simulink model "visodo10"  (Simulink 7.5)
settings: Solver=FixedStepDiscrete  StartTime=0.0  StopTime=220  FixedStep=1  RelTol=1e-3
undefined symbols (not defined in the file): gray, strel
libraries: vipsnks x2, viptextngfix x1, vipmorphops x1
(part 1 of 2)
settings Model: Creator=jfabia02  LastModifiedBy=jfabia02  SimulationMode=external  ExtModeEnableFloating=off  ExtModeArchiveFileName=model_output  ExtModeArchiveDirName=C:\RTtools\VU-RLNX\RLNX\RLNX\Simulink Models
settings RTWCC: SystemTargetFile=rlnx.tlc  GenCodeOnly=on  TemplateMakefile=rlnx_ubuntu.tmf  Description=Linux Real-Time Target  ProcessScript=rlnx_make_rtw_hook
settings CodeAppCC: GenerateComments=off  SimulinkBlockComments=off
settings STFCustomTargetCC: TargetFunctionLibrary=GNU99 (GNU)  ModelReferenceCompliant=off  GeneratePreprocessorConditionals=Disable all  MatFileLogging=on  SystemTargetFile=rlnx.tlc
settings GRTTargetCC: TargetFunctionLibrary=GNU99 (GNU)  ModelReferenceCompliant=off  ParMdlRefBuildCompliant=off  CompOptLevelCompliant=off  ExtMode=on  ExtModeMexArgs='10.0.0.1'
settings CustomProperty: DataType=string  Value=-lm -ldl /matlab_includes/libfreenect/build/lib/libfreenect.so.0.0.1
settings EnumStrPairs: String=PC

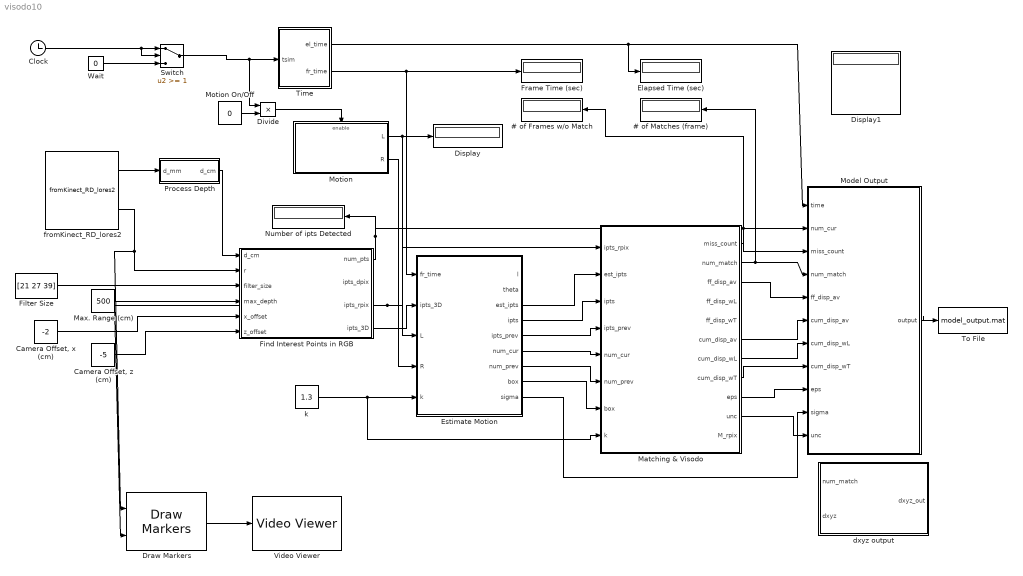
== system visodo10 ==
  # of Frames w/o Match : Display
  # of Matches (frame) : Display
  "Camera Offset, x (cm)" : Constant  Value=-2  OutDataTypeMode=double  OutDataType=fixdt(1, 16)  OutScaling=2^0  OutDataTypeStr=double
  "Camera Offset, z (cm)" : Constant  Value=-5  OutDataTypeMode=double  OutDataType=fixdt(1, 16)  OutScaling=2^0  OutDataTypeStr=double
  Clock : Clock
      settings: Decimation=10
  Display : Display
  Display1 : Display
  Divide : Product  Inputs=**  OutDataType=fixdt(1, 16)  OutScaling=2^-10
  Draw Markers : viptextngfix/Draw Markers  DialogController=vipDDGCreate  DialogControllerArgs=DataTag0  shape=Circle  size=3  fill=off  fillClrSource=Specify via dialog  display=Black  intensity=200  color=[200 255 100]  opacity=0.6  viewport=Entire image  antialiasing=off  inType=Obsolete  imagePorts=One multidimensional signal  prodOutputMode=Binary point scaling  prodOutputWordLength=32  prodOutputFracLength=14  memoryMode=Specify word length  memoryWordLength=16  memoryFracLength=15  roundingMode=Floor  overflowMode=off
  Elapsed Time (sec) : Display
  Estimate Motion : Subsystem
  Filter Size : Constant  Value=[21 27 39]  OutDataType=fixdt(1, 16)  OutScaling=2^0
  Find Interest Points in RGB : Subsystem
  Frame Time (sec) : Display
  Matching & Visodo : Subsystem
  Max. Range (cm) : Constant  Value=500  OutDataType=fixdt(1, 16)  OutScaling=2^0
  Model Output : Stateflow chart  TreatAsAtomicUnit=on
  Motion : Subsystem
  Motion On/Off : Constant  Value=0  OutDataType=fixdt(1, 16)  OutScaling=2^0
  Number of ipts Detected : Display
  Process Depth : Subsystem
  Switch : Switch  Threshold=1  OutDataType=fixdt(1, 16)  OutScaling=2^0
  Time : Subsystem
  To File : ToFile  Filename=model_output.mat  MatrixName=output
  Video Viewer : vipsnks/Video Viewer  DialogControllerArgs=DataTag3  inputType=Obsolete7b  imagePorts=One multidimensional signal  useColorMap=off  colormapValue=gray(256)  specRange=off  minInputVal=0  maxInputVal=255  FigPos=[69 572 410 300]  AxisZoom=on  trueSizedOnce=off  OpenAtMdlStart=on
  Wait : Constant  Value=0  OutDataType=fixdt(1, 16)  OutScaling=2^0
  dxyz output : Stateflow chart  TreatAsAtomicUnit=on
  fromKinect_RD_lores2 : S-Function  FunctionName=fromKinect_RD_lores2  EnableBusSupport=off
      mask Display: image(imread('C:\RTtools\VU-RLNX\RLNX\RLNX\Simulink Models\kinectimage.jpeg'))
  k : Constant  Value=1.3  OutDataType=fixdt(1, 16)  OutScaling=2^0
  wires:
  Find Interest Points in RGB/1(num_pts) -> Number of ipts Detected/1, Model Output/2(num_cur)
  Find Interest Points in RGB/4(ipts_3D) -> Estimate Motion/2(ipts_3D)
  Max. Range (cm)/1 -> Find Interest Points in RGB/4(max_depth)
  Matching & Visodo/2(num_match) -> # of Matches (frame)/1, Model Output/4(num_match)
  Estimate Motion/5(ipts_prev) -> Matching & Visodo/4(ipts_prev)
  Estimate Motion/4(ipts) -> Matching & Visodo/3(ipts)
  Estimate Motion/6(num_cur) -> Matching & Visodo/5(num_cur)
  Estimate Motion/7(num_prev) -> Matching & Visodo/6(num_prev)
  Matching & Visodo/1(miss_count) -> # of Frames w/o Match/1, Model Output/3(miss_count)
  Process Depth/1(d_cm) -> Find Interest Points in RGB/1(d_cm)
  "Camera Offset, x (cm)"/1 -> Find Interest Points in RGB/5(x_offset)
  "Camera Offset, z (cm)"/1 -> Find Interest Points in RGB/6(z_offset)
  Estimate Motion/8(box) -> Matching & Visodo/7(box)
  Estimate Motion/3(est_ipts) -> Matching & Visodo/2(est_ipts)
  Filter Size/1 -> Find Interest Points in RGB/3(filter_size)
  fromKinect_RD_lores2/1 -> Process Depth/1(d_mm)
  fromKinect_RD_lores2/2 -> Find Interest Points in RGB/2(r), Draw Markers/1
  Estimate Motion/9(sigma) -> Model Output/10(sigma)
  Clock/1 -> Switch/1, Switch/2
  Wait/1 -> Switch/3
  Switch/1 -> Time/1(tsim), Divide/1
  Motion On/Off/1 -> Divide/2
  Divide/1 -> Motion/Enable
  Motion/1(L) -> Estimate Motion/3(L), Display/1
  Motion/2(R) -> Estimate Motion/4(R)
  Time/2(fr_time) -> Estimate Motion/1(fr_time), Frame Time (sec)/1
  Time/1(el_time) -> Elapsed Time (sec)/1, Model Output/1(time)
  Model Output/1(output) -> To File/1
  k/1 -> Estimate Motion/5(k), Matching & Visodo/8(k)
  Matching & Visodo/9(eps) -> Model Output/9(eps)
  Find Interest Points in RGB/3(ipts_rpix) -> Matching & Visodo/1(ipts_rpix), Draw Markers/2
  Matching & Visodo/6(cum_disp_av) -> Model Output/6(cum_disp_av)
  Matching & Visodo/7(cum_disp_wL) -> Model Output/7(cum_disp_wL)
  Matching & Visodo/8(cum_disp_wT) -> Model Output/8(cum_disp_wT)
  Matching & Visodo/3(ff_disp_av) -> Model Output/5(ff_disp_av)
  Matching & Visodo/10(unc) -> Model Output/11(unc)
  Draw Markers/1 -> Video Viewer/1

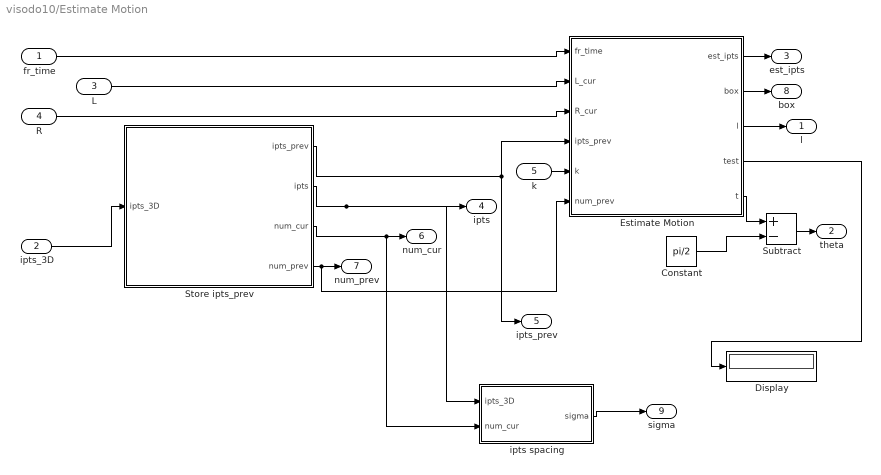
== system visodo10/Estimate Motion ==
  fr_time : Inport
  ipts_3D : Inport  Port=2
  L : Inport  Port=3
  R : Inport  Port=4
  k : Inport  Port=5
  Constant : Constant  Value=pi/2  OutDataType=fixdt(1, 16)  OutScaling=2^0
  Display : Display
  Estimate Motion : Stateflow chart  TreatAsAtomicUnit=on
  Store ipts_prev : Stateflow chart  TreatAsAtomicUnit=on
  Subtract : Sum  Inputs=+-  OutDataType=fixdt(1, 16)  OutScaling=2^-10
  ipts spacing : Stateflow chart  TreatAsAtomicUnit=on
  l : Outport
  theta : Outport  Port=2
  est_ipts : Outport  Port=3
  ipts : Outport  Port=4
  ipts_prev : Outport  Port=5
  num_cur : Outport  Port=6
  num_prev : Outport  Port=7
  box : Outport  Port=8
  sigma : Outport  Port=9  OutDataType=fixdt(1, 16)  OutScaling=2^0
  wires:
  Estimate Motion/1(est_ipts) -> est_ipts/1
  ipts_3D/1 -> Store ipts_prev/1(ipts_3D)
  Store ipts_prev/3(num_cur) -> num_cur/1, ipts spacing/2(num_cur)
  Store ipts_prev/4(num_prev) -> num_prev/1, Estimate Motion/6(num_prev)
  Store ipts_prev/1(ipts_prev) -> ipts_prev/1, Estimate Motion/4(ipts_prev)
  fr_time/1 -> Estimate Motion/1(fr_time)
  L/1 -> Estimate Motion/2(L_cur)
  R/1 -> Estimate Motion/3(R_cur)
  Estimate Motion/2(box) -> box/1
  k/1 -> Estimate Motion/5(k)
  ipts spacing/1(sigma) -> sigma/1
  Store ipts_prev/2(ipts) -> ipts/1, ipts spacing/1(ipts_3D)
  Estimate Motion/3(l) -> l/1
  Subtract/1 -> theta/1
  Estimate Motion/5(t) -> Subtract/1
  Constant/1 -> Subtract/2
  Estimate Motion/4(test) -> Display/1

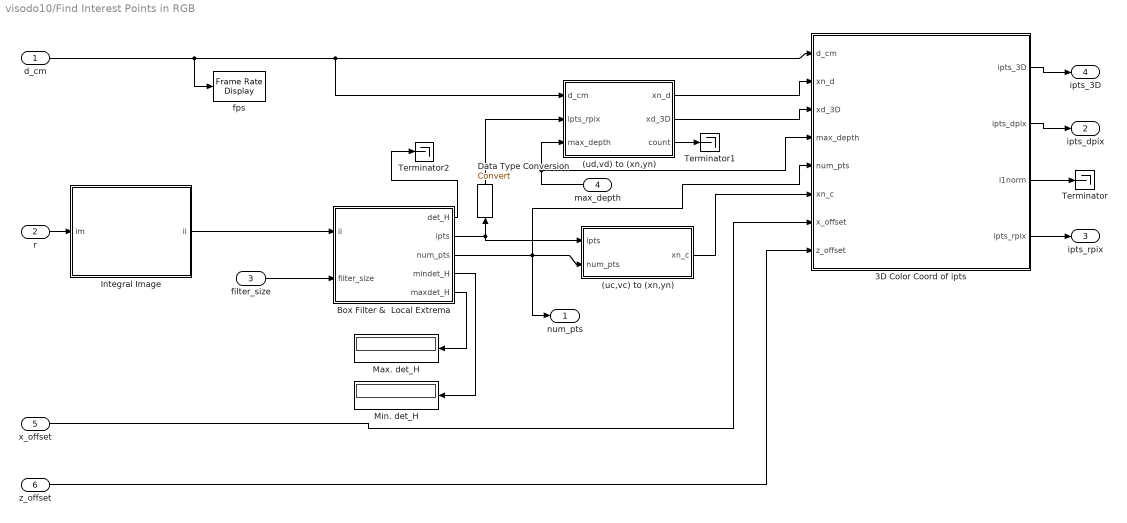
== system visodo10/Find Interest Points in RGB ==
  d_cm : Inport
  r : Inport  Port=2
  filter_size : Inport  Port=3  OutDataType=fixdt(1, 16)  OutScaling=2^0
  max_depth : Inport  Port=4  OutDataType=fixdt(1, 16)  OutScaling=2^0
  x_offset : Inport  Port=5  OutDataType=fixdt(1, 16)  OutScaling=2^0
  z_offset : Inport  Port=6  OutDataType=fixdt(1, 16)  OutScaling=2^0
  (uc,vc) to (xn,yn) : Stateflow chart  TreatAsAtomicUnit=on
  (ud,vd) to (xn,yn) : Stateflow chart  TreatAsAtomicUnit=on
  3D Color Coord of ipts : Stateflow chart  TreatAsAtomicUnit=on
  Box Filter &  Local Extrema : Stateflow chart  TreatAsAtomicUnit=on
  Data Type Conversion : DataTypeConversion  OutDataType=fixdt(1, 16)  OutScaling=2^0
  Integral Image : Stateflow chart  TreatAsAtomicUnit=on
  Max. det_H : Display
  Min. det_H : Display
  Terminator : Terminator
  Terminator1 : Terminator
  Terminator2 : Terminator
  fps : vipsnks/Frame Rate Display  DialogController=vipDDGCreate  DialogControllerArgs=DataTag1  UpdateRate=10
  num_pts : Outport
  ipts_dpix : Outport  Port=2
  ipts_rpix : Outport  Port=3
  ipts_3D : Outport  Port=4
  wires:
  r/1 -> Integral Image/1(im)
  filter_size/1 -> Box Filter &  Local Extrema/2(filter_size)
  Box Filter &  Local Extrema/2(ipts) -> Data Type Conversion/1, (uc,vc) to (xn,yn)/1(ipts)
  Integral Image/1(ii) -> Box Filter &  Local Extrema/1(ii)
  (ud,vd) to (xn,yn)/1(xn_d) -> 3D Color Coord of ipts/2(xn_d)
  (ud,vd) to (xn,yn)/2(xd_3D) -> 3D Color Coord of ipts/3(xd_3D)
  d_cm/1 -> (ud,vd) to (xn,yn)/1(d_cm), 3D Color Coord of ipts/1(d_cm), fps/1
  (uc,vc) to (xn,yn)/1(xn_c) -> 3D Color Coord of ipts/6(xn_c)
  3D Color Coord of ipts/4(ipts_rpix) -> ipts_rpix/1
  Box Filter &  Local Extrema/3(num_pts) -> (uc,vc) to (xn,yn)/2(num_pts), num_pts/1, 3D Color Coord of ipts/5(num_pts)
  max_depth/1 -> (ud,vd) to (xn,yn)/3(max_depth), 3D Color Coord of ipts/4(max_depth)
  x_offset/1 -> 3D Color Coord of ipts/7(x_offset)
  z_offset/1 -> 3D Color Coord of ipts/8(z_offset)
  Box Filter &  Local Extrema/5(maxdet_H) -> Max. det_H/1
  Box Filter &  Local Extrema/4(mindet_H) -> Min. det_H/1
  3D Color Coord of ipts/2(ipts_dpix) -> ipts_dpix/1
  3D Color Coord of ipts/1(ipts_3D) -> ipts_3D/1
  Data Type Conversion/1 -> (ud,vd) to (xn,yn)/2(ipts_rpix)
  3D Color Coord of ipts/3(l1norm) -> Terminator/1
  (ud,vd) to (xn,yn)/3(count) -> Terminator1/1
  Box Filter &  Local Extrema/1(det_H) -> Terminator2/1

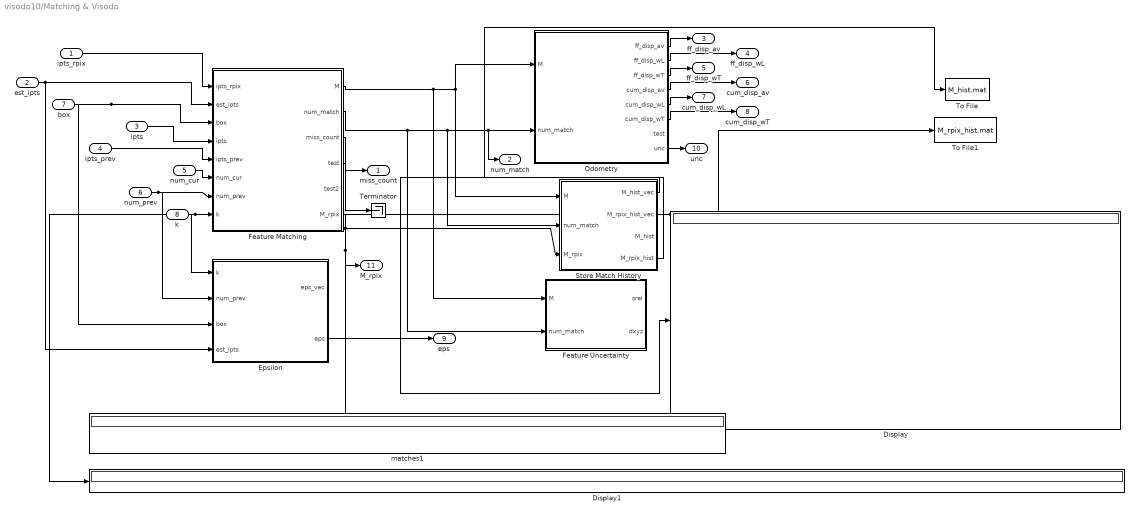
== system visodo10/Matching & Visodo ==
  ipts_rpix : Inport  OutDataType=fixdt(1, 16)  OutScaling=2^0
  est_ipts : Inport  Port=2
  ipts : Inport  Port=3
  ipts_prev : Inport  Port=4
  num_cur : Inport  Port=5
  num_prev : Inport  Port=6
  box : Inport  Port=7
  k : Inport  Port=8  OutDataType=fixdt(1, 16)  OutScaling=2^0
  Display : Display
  Display1 : Display
  Epsilon : Stateflow chart  TreatAsAtomicUnit=on
  Feature Matching : Stateflow chart  TreatAsAtomicUnit=on
  Feature Uncertainty : Stateflow chart  TreatAsAtomicUnit=on
  Odometry : Stateflow chart  TreatAsAtomicUnit=on
  Store Match History : Stateflow chart  TreatAsAtomicUnit=on
  Terminator : Terminator
  To File : ToFile  Filename=M_hist.mat  MatrixName=data
  To File1 : ToFile  Filename=M_rpix_hist.mat  MatrixName=data
  matches1 : Display
  miss_count : Outport
  num_match : Outport  Port=2
  ff_disp_av : Outport  Port=3
  ff_disp_wL : Outport  Port=4
  ff_disp_wT : Outport  Port=5
  cum_disp_av : Outport  Port=6
  cum_disp_wL : Outport  Port=7
  cum_disp_wT : Outport  Port=8
  eps : Outport  Port=9  OutDataType=fixdt(1, 16)  OutScaling=2^0
  unc : Outport  Port=10
  M_rpix : Outport  Port=11
  wires:
  Odometry/1(ff_disp_av) -> ff_disp_av/1
  Odometry/2(ff_disp_wL) -> ff_disp_wL/1
  Feature Matching/1(M) -> Odometry/1(M), Store Match History/1(M), Feature Uncertainty/1(M)
  box/1 -> Epsilon/3(box), Feature Matching/3(box)
  ipts/1 -> Feature Matching/4(ipts)
  ipts_prev/1 -> Feature Matching/5(ipts_prev)
  num_cur/1 -> Feature Matching/6(num_cur)
  num_prev/1 -> Feature Matching/7(num_prev), Epsilon/2(num_prev)
  Feature Matching/2(num_match) -> Feature Uncertainty/2(num_match), num_match/1, Odometry/2(num_match), Store Match History/2(num_match)
  Feature Matching/3(miss_count) -> miss_count/1
  est_ipts/1 -> Epsilon/4(est_ipts), Feature Matching/2(est_ipts)
  k/1 -> Feature Matching/8(k), Epsilon/1(k)
  Epsilon/2(eps) -> eps/1
  Feature Matching/4(test) -> Terminator/1
  ipts_rpix/1 -> Feature Matching/1(ipts_rpix)
  Odometry/6(cum_disp_wT) -> cum_disp_wT/1
  Odometry/5(cum_disp_wL) -> cum_disp_wL/1
  Odometry/4(cum_disp_av) -> cum_disp_av/1
  Odometry/3(ff_disp_wT) -> ff_disp_wT/1
  Feature Matching/6(M_rpix) -> Store Match History/3(M_rpix), M_rpix/1, matches1/1
  Odometry/8(unc) -> unc/1
  Store Match History/1(M_hist_vec) -> To File/1
  Store Match History/2(M_rpix_hist_vec) -> To File1/1, Display1/1
  Store Match History/4(M_rpix_hist) -> Display/1

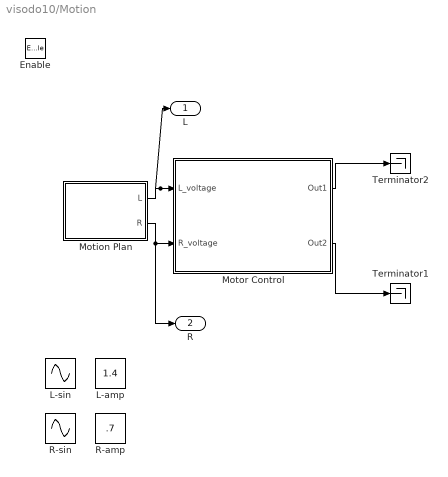
== system visodo10/Motion ==
  Enable : EnablePort
  L-amp : Constant  Value=1.4  OutDataType=fixdt(1, 16)  OutScaling=2^0
  L-sin : Sin  Amplitude=1.2  Bias=2  Frequency=2*pi/60  Phase=-pi/2+.9  Samples=10  SampleTime=1  Offset=0
  Motion Plan : Stateflow chart  TreatAsAtomicUnit=on
  Motor Control : Subsystem
  R-amp : Constant  Value=.7  OutDataType=fixdt(1, 16)  OutScaling=2^0
  R-sin : Sin  Amplitude=1.2  Bias=2  Frequency=2*pi/60  Phase=pi/2+.9  Samples=10  SampleTime=1  Offset=0
  Terminator1 : Terminator
  Terminator2 : Terminator
  L : Outport  OutDataType=fixdt(1, 16)  OutScaling=2^0  InitialOutput=0
  R : Outport  Port=2  OutDataType=fixdt(1, 16)  OutScaling=2^0  InitialOutput=0
  wires:
  Motor Control/2(Out2) -> Terminator1/1
  Motor Control/1(Out1) -> Terminator2/1
  Motion Plan/1(L) -> Motor Control/1(L_voltage), L/1
  Motion Plan/2(R) -> Motor Control/2(R_voltage), R/1

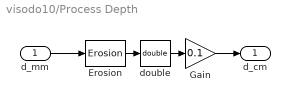
== system visodo10/Process Depth ==
  d_mm : Inport
  Erosion : vipmorphops/Erosion  nhoodsrc=Specify via dialog  strel=strel('square',4)
  Gain : Gain  Gain=0.1  ParameterDataType=fixdt(1, 16)  ParameterScaling=2^0  OutDataTypeMode=double  OutDataType=fixdt(1, 16)  OutScaling=2^0  OutDataTypeStr=double
  double : DataTypeConversion  OutDataTypeMode=double  OutDataType=fixdt(1, 16)  OutScaling=2^0  OutDataTypeStr=double
  d_cm : Outport
  wires:
  Erosion/1 -> double/1
  double/1 -> Gain/1
  d_mm/1 -> Erosion/1
  Gain/1 -> d_cm/1

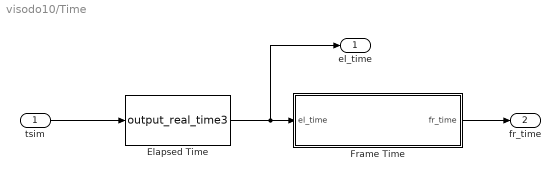
== system visodo10/Time ==
  tsim : Inport  OutDataType=fixdt(1, 16)  OutScaling=2^0
  Elapsed Time : S-Function  FunctionName=output_real_time3  EnableBusSupport=off
  Frame Time : Stateflow chart  TreatAsAtomicUnit=on
  el_time : Outport
  fr_time : Outport  Port=2
  wires:
  tsim/1 -> Elapsed Time/1
  Elapsed Time/1 -> Frame Time/1(el_time), el_time/1
  Frame Time/1(fr_time) -> fr_time/1

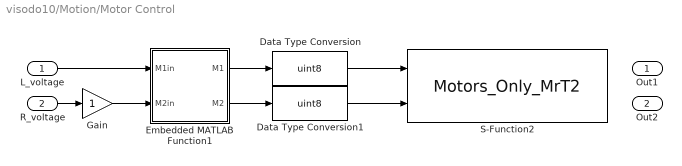
== system visodo10/Motion/Motor Control ==
  L_voltage : Inport
  R_voltage : Inport  Port=2
  Data Type Conversion : DataTypeConversion  OutDataTypeMode=uint8  OutDataType=fixdt(1, 16)  OutScaling=2^0  OutDataTypeStr=uint8
  Data Type Conversion1 : DataTypeConversion  OutDataTypeMode=uint8  OutDataType=fixdt(1, 16)  OutScaling=2^0  OutDataTypeStr=uint8
  Embedded MATLAB Function1 : Stateflow chart  TreatAsAtomicUnit=on
  Gain : Gain  ParameterDataType=fixdt(1, 16)  ParameterScaling=2^0  OutDataType=fixdt(1, 16)  OutScaling=2^0
  S-Function2 : S-Function  FunctionName=Motors_Only_MrT2  EnableBusSupport=off
  Out1 : Outport
  Out2 : Outport  Port=2
  wires:
  ? -> Out2/1
  R_voltage/1 -> Gain/1
  ? -> Out1/1
  L_voltage/1 -> Embedded MATLAB Function1/1(M1in)
  Gain/1 -> Embedded MATLAB Function1/2(M2in)
  Data Type Conversion1/1 -> S-Function2/2
  Data Type Conversion/1 -> S-Function2/1
  Embedded MATLAB Function1/2(M2) -> Data Type Conversion1/1
  Embedded MATLAB Function1/1(M1) -> Data Type Conversion/1

== matlab function dxyz output ==
  data: num_match input double; dxyz input double; dxyz_out output double
%%%%%%%%%%%%%%%%%%%%%%%%
%%%%%%%%%%%%%%%%%%%%%%%%
function dxyz_out = dxyz_output(num_match,dxyz)
% generic function to package multiple signals for output to .mat file


dxyz_out = zeros(601 ,1);
% % dxyz_out(1,1) = num_match;
% % dxyz_out(2:101,1) = dxyz(1,1:100);
% % dxyz_out(102:201,1) = dxyz(2,1:100);
% % dxyz_out(202:301,1) = dxyz(3,1:100);
% % dxyz_out(302:401,1) = dxyz(4,1:100);
% % dxyz_out(402:501,1) = dxyz(5,1:100);
% % dxyz_out(502:601,1) = dxyz(6,1:100);

== matlab function Model Output ==
  data: time input double; num_cur input double; miss_count input double; num_match input double; ff_disp_av input double; cum_disp_av input double; cum_disp_wL input double; cum_disp_wT input double; eps input double; sigma input double; output output double; unc input double
%%%%%%%%%%%%%%%%%%%%%%%%
%%%%%%%%%%%%%%%%%%%%%%%%
% code to record 3D displacements of features
function output = model_output(time, num_cur, miss_count, num_match, ff_disp_av, cum_disp_av, cum_disp_wL,cum_disp_wT,eps,sigma,unc)
% generic function to package multiple signals for output to .mat file


output = zeros(24 ,1);
output(1,1) = time;
output(2,1) = num_cur;
output(3,1) = num_match;
output(4,1) = miss_count;
output(5:8,1) = ff_disp_av(1:4);
output(9:12,1) = cum_disp_av(1:4);
output(13:16,1) = cum_disp_wL(1:4);
output(17:20,1) = cum_disp_wT(1:4);
output(21,1) = sigma;
output(22,1) = eps;
output(23:24,1)= unc;


%%%%%%%%%%%%%%%%%%%%%%%
%%%%%%%%%%%%%%%%%%%%%%%

== matlab function Find Interest Points in RGB/Integral Image ==
  data: im input double; ii output double
function ii = integral_image(im)
% function input is image, im
% output is integral image, ii
im = double(im);
height = size(im,1);
width = size(im,2);
ii = double(zeros(height, width));
col_sum = zeros(height,1);

ii(1,1) = double(im(1,1));
% first column
for j = 2:height
    ii(j,1) = im(j,1) + ii(j-1,1);
end
% first row
for i = 2:width
    ii(1,i) = im(1,i) + ii(1, i-1);
end
% rest of image
for i = 2:width
    col_sum(1,1) = im(1,i);
    for j = 2:height
        col_sum(j,1) = im(j,i) + col_sum(j-1,1);
        ii(j,i) = col_sum(j,1) + ii(j,i-1);
    end
end

== matlab function Matching & Visodo/Epsilon ==
  data: eps_vec output double; k input double; num_prev input double; eps output double; box input double; est_ipts input double
function [eps_vec, eps] = calc_eps(k, num_prev, box, est_ipts)
% function calculates epsilon for each ipts


%%%%%%%%%%%%%%%%%%%%%%%%%%%%%%%%%%%%%%%%%
%%%%%%%%%%%%%%%%%%%%%%%%%%%%%%%%%%%%%%%%%
% alternate epsilon based on feature closest to z=100cm
eps_vec=zeros(1,100);
eps=0;
if num_prev>0
    ave_depth=median(est_ipts(3,1:num_prev));
    [val,ind]=min(abs(est_ipts(3,1:num_prev)-ave_depth));
    xh=est_ipts(1,ind);
    yh=est_ipts(2,ind);
    zh=est_ipts(3,ind);
    c1x=box(1,ind);
    c1z=box(4,ind);
    cyt=box(6,ind);
    eps=sqrt((c1x-xh)^2+(c1z-zh)^2+(cyt-yh)^2);
end

== matlab function Find Interest Points in RGB/Box Filter & Local Extrema ==
  data: det_H output double; ipts output double; ii input double; filter_size input double; num_pts output double; mindet_H output double; maxdet_H output double

function [det_H, ipts, num_pts, mindet_H, maxdet_H]  = box_filter(ii, filter_size)
% input is integral image calculated in 'Integral Image'
% ipts across 3 scales:
%   - either 15, 27, 39 
%   - or 27, 39, 51

%%%%%%%%%%%%%%%%%%%%%%%%%%%%%%%%%%%%%%%%%%%%%%%%%%%%%%%%%%%%%%%%%%%%%%%
pos_thres = 100;  % use this threshold to fire on high-contrast areas
neg_thres = -100; % det_H range is generally not symmetric about zero
max_num_ipts = 100; %%%%% 
min_sep = 3; %% minimum separation, in pixels, between adjacent ipts
%%%%%%%%%%%%%%%%%%%%%%%%%%%%%%%%%%%%%%%%%%%%%%%%%%%%%%%%%%%%%%%%%%%%%%%


h = size(ii,1);
w = size(ii,2);
det_H = zeros(h,w);
mindet_H = 0;
maxdet_H = 0;

ipts = uint16(zeros(2,max_num_ipts));
num_pts = 0;
count = 0;
    
Dyy = zeros(h,w);
Dxx = zeros(h,w);
Dxy = zeros(h,w);    

persistent fc area fs2d3 fc1 area1 fs1d3 fc3 area3 fs3d3
if isempty(fc)
    % calculate related filter dimensions
    fc = round(filter_size(2)/2);
    area = filter_size(2)*filter_size(2);
    fs2d3 = (filter_size(2)/3);

    fc1 = round(filter_size(1)/2);
    area1 = filter_size(1)*filter_size(1);
    fs1d3 = (filter_size(1)/3);

    fc3 = round(filter_size(3)/2);
    area3 = filter_size(3)*filter_size(3);
    fs3d3 = (filter_size(3)/3);
end

for i = fc3+1:(w-fc3)
    for j = fc3+1:(h-fc3)
        % reference points for computing response from integral image
        % o's are Dyy pts, c's are Dxx pts, q's are Dxy pts.
        oj1 = j - fc;
        oi1 = i - (fs2d3); oi2 = oi1; oi3 = oi1; oi4 = oi1;
        oj2 = j - fc + (fs2d3);        
        oj3 = j + fc - (fs2d3)-1;        
        oj4 = j + fc - 1;        
        oj5 = oj1; oj6 = oj2; oj7 = oj3; oj8 = oj4;
        oi5 = i + (fs2d3) -1; oi6 = oi5; oi7 = oi5; oi8 = oi5;
        Dyy(j,i) = 2*(ii(oj7,oi7) - ii(oj6,oi6) -ii(oj3,oi3) + ii(oj2,oi2))...
                   - (ii(oj6,oi6) - ii(oj5,oi5) - ii(oj2,oi2) + ii(oj1,oi1))...
                   - (ii(oj8,oi8) - ii(oj7,oi7) - ii(oj4,oi4) + ii(oj3,oi3));

        ci1 = i - fc;
        cj1 = j - (fs2d3); cj2 = cj1; cj3 = cj1; cj4 = cj1;
        ci2 = i - fc + (fs2d3);        
        ci3 = i + fc - (fs2d3)-1;        
        ci4 = i + fc - 1;        
        ci5 = ci1; ci6 = ci2; ci7 = ci3; ci8 = ci4;
        cj5 = j + (fs2d3) -1; cj6 = cj5; cj7 = cj5; cj8 = cj5;
        Dxx(j,i) = 2*(ii(cj7,ci7) - ii(cj6,ci6) -ii(cj3,ci3) + ii(cj2,ci2))...
                   - (ii(cj6,ci6) - ii(cj5,ci5) - ii(cj2,ci2) + ii(cj1,ci1))...
                   - (ii(cj8,ci8) - ii(cj7,ci7) - ii(cj4,ci4) + ii(cj3,ci3));

        qi1 = i-(fs2d3)-1; qi2 = qi1; qi3 = qi1; qi4=qi1;
        qi5 = i-1; qi6=qi5; qi7=qi5; qi8=qi5;
        qi9 = i; qi10 = i; qi11=i; qi12=i;
        qi13 = i+(fs2d3); qi14=qi13; qi15=qi13; qi16=qi13;
        qj1 = j-(fs2d3)-1; qj5=qj1; qj9=qj1; qj13=qj1;
        qj2 = j-1; qj6=qj2; qj10=qj2; qj14=qj2;
        qj3=j; qj7=j; qj11=j; qj15=j;
        qj4=j+(fs2d3); qj8=qj4; qj12=qj4; qj16=qj4;
        Dxy(j,i) = (ii(qj8,qi8)-ii(qj7,qi7)-ii(qj4,qi4)+ii(qj3,qi3))...
                  + (ii(qj14,qi14)-ii(qj13,qi13)-ii(qj10,qi10)+ii(qj9,qi9))...
                  - (ii(qj6,qi6)-ii(qj5,qi5)-ii(qj2,qi2)+ii(qj1,qi1))...
                  -( ii(qj16,qi16)-ii(qj15,qi15)-ii(qj12,qi12)+ii(qj11,qi11));

        det_H(j,i) = ((Dyy(j,i) * Dxx(j,i)) - (0.81*Dxy(j,i)*Dxy(j,i)))/(area*area);
        if det_H(j,i)>maxdet_H
            maxdet_H = det_H(j,i);
        elseif det_H(j,i)<mindet_H
            mindet_H = det_H(j,i);
        end
    end % j
end % i

% find local extrema 
for i = fc+1:(w-fc)
    for j = fc+1:(h-fc)
        if count < max_num_ipts && i>=fc+3 && j>=fc+3
            p = (det_H(j,i));
            t1 = (det_H(j-1,i-1));
            t2 = (det_H(j,i-1));
            t3 = (det_H(j+1,i-1));
            t4 = (det_H(j-1,i));
            t5 = (det_H(j+1,i));
            t6 = (det_H(j-1,i+1));
            t7 = (det_H(j,i+1));
            t8 = (det_H(j+1,i+1));

            if ((p>pos_thres && p>t1 && p>t2 && p>t3 && p>t4 ...
               && p>t5 && p>t6 && p>t7 && p>t8) || ...
               (p<neg_thres && p<t1 && p<t2 && p<t3 && p<t4 ...
               && p<t5 && p<t6 && p<t7 && p<t8)) 
                count = count +1;
                ipts(:,count) = [j;i];

                % delete ipts if too close to previous ipts
                if count>1 
                    flag=0;
                    for n=1:count-1
                        prox=abs(int16(ipts(1,n))-int16(ipts(1,count))) ...
                           + abs(int16(ipts(2,n))-int16(ipts(2,count)));
                       if prox<=min_sep && flag==0;
                            ipts(:,count) = [0;0]; 
                            count =count-1;
                            flag=1; 
                       end
                    end
                end
% %             end
            % at this point, have detected ipts in middle band
            % now, need to check against bottom and top bands
            det_H1=0; Dxx1=0; Dyy1=0; Dxy1=0;
            det_H3=0; Dxx3=0; Dyy3=0; Dxy3=0;

                % build det_H for bottom band, f=1
                oj1 = j - fc1;
                oi1 = i - (fs1d3); oi2 = oi1; oi3 = oi1; oi4 = oi1;
                oj2 = j - fc1 + (fs1d3);        
                oj3 = j + fc1 - (fs1d3)-1;        
                oj4 = j + fc1 - 1;        
                oj5 = oj1; oj6 = oj2; oj7 = oj3; oj8 = oj4;
                oi5 = i + (fs1d3) -1; oi6 = oi5; oi7 = oi5; oi8 = oi5;
                Dyy1 = 2*(ii(oj7,oi7) - ii(oj6,oi6) -ii(oj3,oi3) + ii(oj2,oi2))...
                           - (ii(oj6,oi6) - ii(oj5,oi5) - ii(oj2,oi2) + ii(oj1,oi1))...
                           - (ii(oj8,oi8) - ii(oj7,oi7) - ii(oj4,oi4) + ii(oj3,oi3));

                ci1 = i - fc1;
                cj1 = j - (fs1d3); cj2 = cj1; cj3 = cj1; cj4 = cj1;
                ci2 = i - fc1 + (fs1d3);        
                ci3 = i + fc1 - (fs1d3)-1;        
                ci4 = i + fc1 - 1;        
                ci5 = ci1; ci6 = ci2; ci7 = ci3; ci8 = ci4;
                cj5 = j + (fs1d3) -1; cj6 = cj5; cj7 = cj5; cj8 = cj5;
                Dxx1 = 2*(ii(cj7,ci7) - ii(cj6,ci6) -ii(cj3,ci3) + ii(cj2,ci2))...
                           - (ii(cj6,ci6) - ii(cj5,ci5) - ii(cj2,ci2) + ii(cj1,ci1))...
                           - (ii(cj8,ci8) - ii(cj7,ci7) - ii(cj4,ci4) + ii(cj3,ci3));

                qi1 = i-(fs1d3)-1; qi2 = qi1; qi3 = qi1; qi4=qi1;
                qi5 = i-1; qi6=qi5; qi7=qi5; qi8=qi5;
                qi9 = i; qi10 = i; qi11=i; qi12=i;
                qi13 = i+(fs1d3); qi14=qi13; qi15=qi13; qi16=qi13;
                qj1 = j-(fs1d3)-1; qj5=qj1; qj9=qj1; qj13=qj1;
                qj2 = j-1; qj6=qj2; qj10=qj2; qj14=qj2;
                qj3=j; qj7=j; qj11=j; qj15=j;
                qj4=j+(fs1d3); qj8=qj4; qj12=qj4; qj16=qj4;
                Dxy1 = (ii(qj8,qi8)-ii(qj7,qi7)-ii(qj4,qi4)+ii(qj3,qi3))...
                          + (ii(qj14,qi14)-ii(qj13,qi13)-ii(qj10,qi10)+ii(qj9,qi9))...
                          - (ii(qj6,qi6)-ii(qj5,qi5)-ii(qj2,qi2)+ii(qj1,qi1))...
                          -( ii(qj16,qi16)-ii(qj15,qi15)-ii(qj12,qi12)+ii(qj11,qi11));

                det_H1 = ((Dyy1 * Dxx1) - (0.81*Dxy1*Dxy1))/(area1*area1);

                % build det_H for top band, f=3
                oj1 = j - fc3;
                oi1 = i - (fs3d3); oi2 = oi1; oi3 = oi1; oi4 = oi1;
                oj2 = j - fc3 + (fs3d3);        
                oj3 = j + fc3 - (fs3d3)-1;        
                oj4 = j + fc3 - 1;        
                oj5 = oj1; oj6 = oj2; oj7 = oj3; oj8 = oj4;
                oi5 = i + (fs3d3) -1; oi6 = oi5; oi7 = oi5; oi8 = oi5;
                Dyy3 = 2*(ii(oj7,oi7) - ii(oj6,oi6) -ii(oj3,oi3) + ii(oj2,oi2))...
                           - (ii(oj6,oi6) - ii(oj5,oi5) - ii(oj2,oi2) + ii(oj1,oi1))...
                           - (ii(oj8,oi8) - ii(oj7,oi7) - ii(oj4,oi4) + ii(oj3,oi3));

                ci1 = i - fc3;
                cj1 = j - (fs3d3); cj2 = cj1; cj3 = cj1; cj4 = cj1;
                ci2 = i - fc3 + (fs3d3);        
                ci3 = i + fc3 - (fs3d3)-1;        
                ci4 = i + fc3 - 1;        
                ci5 = ci1; ci6 = ci2; ci7 = ci3; ci8 = ci4;
                cj5 = j + (fs3d3) -1; cj6 = cj5; cj7 = cj5; cj8 = cj5;
                Dxx3 = 2*(ii(cj7,ci7) - ii(cj6,ci6) -ii(cj3,ci3) + ii(cj2,ci2))...
                           - (ii(cj6,ci6) - ii(cj5,ci5) - ii(cj2,ci2) + ii(cj1,ci1))...
                           - (ii(cj8,ci8) - ii(cj7,ci7) - ii(cj4,ci4) + ii(cj3,ci3));

                qi1 = i-(fs3d3)-1; qi2 = qi1; qi3 = qi1; qi4=qi1;
                qi5 = i-1; qi6=qi5; qi7=qi5; qi8=qi5;
                qi9 = i; qi10 = i; qi11=i; qi12=i;
                qi13 = i+(fs3d3); qi14=qi13; qi15=qi13; qi16=qi13;
                qj1 = j-(fs3d3)-1; qj5=qj1; qj9=qj1; qj13=qj1;
                qj2 = j-1; qj6=qj2; qj10=qj2; qj14=qj2;
                qj3=j; qj7=j; qj11=j; qj15=j;
                qj4=j+(fs3d3); qj8=qj4; qj12=qj4; qj16=qj4;
                Dxy3 = (ii(qj8,qi8)-ii(qj7,qi7)-ii(qj4,qi4)+ii(qj3,qi3))...
                          + (ii(qj14,qi14)-ii(qj13,qi13)-ii(qj10,qi10)+ii(qj9,qi9))...
                          - (ii(qj6,qi6)-ii(qj5,qi5)-ii(qj2,qi2)+ii(qj1,qi1))...
                          -( ii(qj16,qi16)-ii(qj15,qi15)-ii(qj12,qi12)+ii(qj11,qi11));

                det_H3 = ((Dyy3 * Dxx3) - (0.81*Dxy3*Dxy3))/(area3*area3);

                % delete if ipts is not max relative to bottom and top bands
                if (abs(p)>abs(det_H1) && abs(p)>abs(det_H3))
                    continue
                else
                    ipts(:,count) = [0;0]; 
                    count =count-1;      
                end
            end
        end % if count < max_num_ipts
    end % j
end % i
 
num_pts = count; % number of ipts found...could be less than max_num_ipts

== matlab function Matching & Visodo/Odometry ==
  data: M input double; ff_disp_av output double; ff_disp_wL output double; ff_disp_wT output double; cum_disp_av output double; cum_disp_wL output double; cum_disp_wT output double; num_match input double; test output double; unc output double
function [ff_disp_av, ff_disp_wL, ff_disp_wT, cum_disp_av, cum_disp_wL, cum_disp_wT, test, unc] = odometry(M, num_match)
% function takes matrix of matches, 'M', and calculates the 
%   - frame-to-frame displacement (straight average and weighted)
%   - cumulative displacement (straight average and weighted)
% Displacement format is: [delta_x 
%                         [delta_z
%                         [l2
%                         [delta_h ]

persistent cum_disp_av_pers cum_disp_wL_pers cum_disp_wT_pers 
if isempty(cum_disp_av_pers)
    cum_disp_av_pers = [0;0;0;0];
    cum_disp_wL_pers = [0;0;0;0];
    cum_disp_wT_pers = [0;0;0;0];

end
ff_disp_av = [0;0;0;0];
ff_disp_wL = [0;0;0;0];
ff_disp_wT = [0;0;0;0];

n = num_match; 
if n==0 %no actual matches, M(:,1)=est_ipts;
    n=1;
end

ff_disp_vec3 = zeros(4,100);
cum_disp_av = zeros(4,1);
cum_disp_wL = zeros(4,1);
cum_disp_wT = zeros(4,1);

test=zeros(4,100);
unc=[0;0];
sL=zeros(1,100);
sT=zeros(1,100);
sT2=zeros(1,100);
disp_av = zeros(4,1);
disp_wL = zeros(4,1);
disp_wT = zeros(4,1);
sum_wL = 0;
sum_wT = 0;

for i=1:n
        xp = M(1,i); % correct for offset of camera from axle
        zp = M(3,i);
        xc = M(4,i);         
        zc = M(6,i);

        % 2DOF model
% %         L2 = -zc + sqrt(xp*xp+zp*zp-xc*xc); 
% %         A = [xp -zp;zp xp];
% %         c = [xc; (zc+L2)];
% %         b=A\c;
% %         theta = atan2(b(1),b(2));
% %         dh=theta-1.5708; %change in heading...positive for CCW, negative for CW
% %         delta_x = L2*cos(theta);
% %         delta_z = L2*sin(theta);
% %         ff_disp_vec2(1:4,i) = [delta_x;delta_z;L2;dh;];
        
        % 3DOF model
        theta1=atan2(zp+zc,xp-xc);
        theta2=theta1-pi;
        theta12=theta1+theta2;
        c12=cos(theta12);
        s12=sin(theta12);
        c1=cos(theta1);
        s1=sin(theta1);
% %         L3=(xp-c12*xc+s12*zc)/c1;
        L3=(zp-s12*xc-c12*zc)/s1;
        delta_x3=L3*cos(theta1);
        delta_z3=L3*sin(theta1);
        ff_disp_vec3(1:4,i)=[delta_x3;delta_z3;L3;theta12];
        
        % calculate uncertainties for weighting average solution
% %         sL(1,i)=((abs(L2+zc)^-1)*sqrt(2e-4*(xc^4+xp^4)+2e-10*(zp^6+zc^4*(L2+zc)^2))); %% 2DOF solution
               
% %         N=xc*xp+zp*(L2+zc);
% %         D=xp*(L2+zc)-xc*zp;
        sxp2=2e-4*xp^2;
        sxc2=2e-4*xc^2;
        szp2=2e-10*zp^4;
        szc2=2e-10*zc^4;
% %         sT(1,i)=(D^2+N^2)^-1*sqrt((xp*D+zp*N)^2*sxc2+(xc*D-(L2+zc)*N)^2*sxp2 ... %% 2DOF solution
% %             +(zp*D-xp*N)^2*szc2+((L2+zc)*D+xc*N)^2*szp2+(zp*D-xp*N)^2*sL(1,i)^2);
        
        sT(1,i)=(1.4142*abs(xp-xc)/((xp-xc)^2+(zp+zc)^2))*sqrt(szp2+szc2+tan(theta1)^2*(sxp2+sxc2)) + 1e-10;  %% 1e-10 added to avoid singularlity in weighted average
% %         sT2(1,i)=(1.4142)*(1/(1+tan(theta1)^2))*(1/abs(xp-xc))*sqrt(szp2+szc2+tan(theta1)^2*(sxp2+sxc2)) + 1e-10;  %% 1e-10 added to avoid singularlity in weighted average
% %         sL(1,i)=(1/c1)*sqrt(sxp2+s12^2*szc2+c12^2*sxc2+(c12*zc+s12*xc)^2*sT(1,i)^2+s1^2*L3^2*(sT(1,i)/1.4142)^2);
        sL(1,i)=abs(1/s1)*sqrt(szp2+s12^2*sxc2+c12^2*szc2+(-c12*xc+s12*zc)^2*sT(1,i)^2+c1^2*L3^2*(sT(1,i)/1.4142)^2);
        test(1:2,i)=[sT(1,i);sT2(1,i)];        
end % i

if n>1
    sL_max=max(sL(1:n));
    sL_min=min(sL(1:n));
    sT_max=max(sT(1:n));
    sT_min=min(sT(1:n));

    for i=1:n
        wL=(sL(i).^-1-sL_max.^-1)./(sL_min.^-1-sL_max.^-1);
        wT=(sT(i).^-1-sT_max.^-1)./(sT_min.^-1-sT_max.^-1);
        if isnan(wL)
            wL=0;
        elseif isnan(wT)
            wT=0;
        end
        disp_av=ff_disp_vec3(1:4,i) + disp_av;
        disp_wL=wL.*ff_disp_vec3(1:4,i) + disp_wL;
        disp_wT=wT.*ff_disp_vec3(1:4,i) + disp_wT;
        sum_wL=sum_wL+wL;
        sum_wT=sum_wT+wT;
% %         test(1:4,i)=[sT(1,i);sT_min;sT_max;wT];
    end
        ff_disp_av = disp_av./n;
        ff_disp_wL = disp_wL./sum_wL;
        ff_disp_wT = disp_wT./sum_wT;
else
    ff_disp_av=ff_disp_vec3(:,1);
    ff_disp_wL=ff_disp_vec3(:,1);
    ff_disp_wT=ff_disp_vec3(:,1);
end


if isnan(ff_disp_av(1,1))
    ff_disp_av = [0;0;0;0];
end
if isnan(ff_disp_wL(1,1))
    ff_disp_wL = [0;0;0;0];
end
if isnan(ff_disp_wT(1,1))
    ff_disp_wT = [0;0;0;0];
end

    
% calculate cumulative visodo
%% based on straight average...
cum_disp_av(3,1) = cum_disp_av_pers(3,1) + ff_disp_av(3,1); % L
cum_disp_av(4,1) = cum_disp_av_pers(4,1) + ff_disp_av(4,1); % dh
cum_disp_av(1,1)=cum_disp_av_pers(1,1) - (ff_disp_av(3,1))*sin(cum_disp_av_pers(4,1)+(ff_disp_av(4,1))/2); % cum x
cum_disp_av(2,1)=cum_disp_av_pers(2,1) + (ff_disp_av(3,1))*cos(cum_disp_av_pers(4,1)+(ff_disp_av(4,1))/2); % cum z

%% weighted by uncertainty in L...
cum_disp_wL(3,1) = cum_disp_wL_pers(3,1) + ff_disp_wL(3,1); % L
cum_disp_wL(4,1) = cum_disp_wL_pers(4,1) + ff_disp_wL(4,1); % dh
cum_disp_wL(1,1)=cum_disp_wL_pers(1,1) - (ff_disp_wL(3,1))*sin(cum_disp_wL_pers(4,1)+(ff_disp_wL(4,1))/2); % cum x
cum_disp_wL(2,1)=cum_disp_wL_pers(2,1) + (ff_disp_wL(3,1))*cos(cum_disp_wL_pers(4,1)+(ff_disp_wL(4,1))/2); % cum z

%% weighted by uncertainty in Theta...
cum_disp_wT(3,1) = cum_disp_wT_pers(3,1) + ff_disp_wT(3,1); % L
cum_disp_wT(4,1) = cum_disp_wT_pers(4,1) + ff_disp_wT(4,1); % dh
cum_disp_wT(1,1)=cum_disp_wT_pers(1,1) - (ff_disp_wT(3,1))*sin(cum_disp_wT_pers(4,1)+(ff_disp_wT(4,1))/2); % cum x
cum_disp_wT(2,1)=cum_disp_wT_pers(2,1) + (ff_disp_wT(3,1))*cos(cum_disp_wT_pers(4,1)+(ff_disp_wT(4,1))/2); % cum z

% store persistent variables
cum_disp_av_pers = cum_disp_av;
cum_disp_wL_pers = cum_disp_wL;
cum_disp_wT_pers = cum_disp_wT;

unc(1:2,1)=[mean(sL(1:n));mean(sT(1:n))];

== matlab function Estimate Motion/Estimate Motion ==
  data: fr_time input double; L_cur input double; R_cur input double; est_ipts output double; ipts_prev input double; box output double; k input double; l output double; test output double; t output double; num_prev input double
function [est_ipts, box, l, test, t]  = est_mot(fr_time, L_cur, R_cur, ipts_prev, k, num_prev)
% function estimates the current of each previous ipts_3D based on motion command
% sent to motors...for use as 'exp_val' in 'Feature Matching' block

% 'motion' has 6 settings:
% 1 = stop
% 2 = rotate CCW
% 3 = rotate CW
% 4 = move forward
% 5 = reverse
% 6 = terminate program
persistent L_pers R_pers
if isempty(L_pers)
    L_pers=0;
    R_pers=0;
end


max_num_ipts = 100; %%%%% must be same for 'find_local_extrema', 'uc_to_xk' and 'ipts_to_3Dcolor'
alpha=0.008; % angular uncertainty
delta=.8; % linear uncertainty

test=0;

est_ipts = zeros(3,max_num_ipts);
box = zeros(7,max_num_ipts); % contains corners of matching region, [c1x,c1z,c2x,c2z,...].

%% build motion estimate vector, x_hat=[l_hat;theta_hat]
if L_cur~=L_pers
    L=0.5*(L_cur+L_pers);
else
    L=L_cur;
end
if R_cur~=R_pers
    R=0.5*(R_cur+R_pers);
else
    R=R_cur;
end
L_pers=L_cur;
R_pers=R_cur;
Vl=L*4.5; % lin. velocity of left wheel
Vr=R*4.5; % lin. vel of right wheel
v=0.5*(Vl+Vr); % lin vel of center of robot
w=(Vr-Vl)/31.5; % ang vel of center of robot (2*half-axle=31.5)

l=v*fr_time;
t=1.5708+w*fr_time;

%%%%%%%%%%%%%%%
%% uncomment below to use actual_disp as motion estimate
% % l=est_lin_vel;
% % t=est_ang_vel+1.5708;
%%%%%%%%%%%%%%%

for i=1:max_num_ipts
    rx=0;
    rz=0;
% %     est_ipts(1:3,i) = [sin(t) 0 -cos(t); 0 1 0; cos(t) 0 sin(t)]*(ipts_prev(:,i))-[0;0;l]; %%2DOF forward kin
    dh=w*fr_time;
    t1=(dh+pi)/2;
    c12=cos(dh);
    s12=sin(dh);
    s1=sin(t1);
    c1=cos(t1);
    xp=ipts_prev(1,i);
    yp=ipts_prev(2,i);
    zp=ipts_prev(3,i);
    est_ipts(1:3,i) = [c12 0 s12;0 1 0; -s12 0 c12]*[xp-l*c1; yp; zp-l*s1]; %% 3DOF forward solution
    xh=est_ipts(1,i);
    yh=est_ipts(2,i);
    zh=est_ipts(3,i);
% %     rx=0.006*est_ipts(3,i) + alpha*(est_ipts(3,i)+l);
% %     rz=1.44e-5*est_ipts(3,1)^2 +(est_ipts(1,i)*alpha+delta);
    
    sx=abs(k*1.4e-2*xh);
    sy=abs(k*2*2.3e-2*yh);
    sz=abs(k*1.44e-5*zh*zh);
    
    if xh>=0
        ex_l=k*abs(xh*(cos(-alpha)-1)+zh*sin(-alpha)+l*sin(-alpha));
        ex_r=k*abs(xh*(cos(alpha)-1)+zh*sin(alpha)+l*sin(alpha));
        
    else
        ex_r=k*abs(xh*(cos(-alpha)-1)+zh*sin(-alpha)+l*sin(-alpha));
        ex_l=k*abs(xh*(cos(alpha)-1)+zh*sin(alpha)+l*sin(alpha));
        
    end
    
    left=xh-sx-ex_l;
    right=xh+sx+ex_r;
    top_y=max([yh+sy yh-sy]);
    bot_y=min([yh+sy yh-sy]);
    m=2*xh*sin(alpha)/(left-right);
    ez2=k*(zh*(cos(alpha)-1)-xh*sin(alpha)+l*(cos(alpha)-1)+delta);
    ez4=k*(zh*(cos(alpha)-1)-xh*sin(alpha)+l*(cos(alpha)-1)-delta);
    z2=zh+sz+ez2;
    z4=zh-sz+ez4;
    
    
% %     ex1=k*(xh*(cos(alpha)-1)+zh*sin(alpha)+l*sin(alpha));
% %     ez1=k*(zh*(cos(alpha)-1)-xh*sin(alpha)+l*(cos(alpha)-1)-delta);
% %     ex2=ex1;
% %     ez2=k*(zh*(cos(alpha)-1)-xh*sin(alpha)+l*(cos(alpha)-1)+delta);
% %     ex3=k*(xh*(cos(-alpha)-1)+zh*sin(-alpha)+l*sin(-alpha));
% %     ez3=k*(zh*(cos(-alpha)-1)-xh*sin(-alpha)+l*(cos(-alpha)-1)+delta);
% %     ex4=ex3;
% %     ez4=k*(zh*(cos(-alpha)-1)-xh*sin(-alpha)+l*(cos(-alpha)-1)-delta);
    
    box(1:7,i)=[left;...
                right;...
                m;...
                z2;...
                z4;...
                top_y;...
                bot_y];
       
end

% % test=mean(abs(box(9,1:num_prev)-box(10,1:num_prev)));

== matlab function Find Interest Points in RGB/(uc,vc) to (xn,yn) ==
  data: ipts input double; num_pts input double; xn_c output double
function xn_c  = uc_to_xn(ipts, num_pts)
% function builds LUT for xk and...
% converts ipts in (uc, vc) from 'find local extrema' into (xn, yn)


persistent xk_LUT x_inc y_inc x_init x_fin y_init y_fin uc0 vc0 fxc fyc LUT_x_steps LUT_y_steps
if isempty(xk_LUT)
    %%%% Define grid for xk_LUT %%%%%%%%
    x_inc = .01; % frame rate very sensitive to these values
    y_inc = .02;
    x_init = -0.58;
    x_fin = 0.52;
    y_init = -0.36;
    y_fin = 0.13;
    %%%%%%%%%%%%%%%%%%%%%%%%%%%%%%%%%%%%
    
    
    k1=.1925; k2=-.384; k3=.0022; k4=.0056;
    x = x_init:x_inc:x_fin;
    y = y_init:y_inc:y_fin;

    [xn, yn] = meshgrid(x,y);

    xk=xn.*(1+k1.*(xn.^2+yn.^2)+k2.*(xn.^4+yn.^4+2*xn.^2.*yn.^2)) + 2*k3.*xn.*yn + k4.*(3.*xn.^2+yn.^2);
    yk=yn.*(1+k1.*(xn.^2+yn.^2)+k2.*(xn.^4+yn.^4+2*xn.^2.*yn.^2)) + 2*k4.*xn.*yn + k3.*(3.*yn.^2+xn.^2);

    xk_LUT = zeros(size(xk,1),size(xk,2),2);
    xk_LUT(:,:,1) = xk;
    xk_LUT(:,:,2) = yk;
    
    % rgb intrinsics
    uc0 = 318.2174; vc0 = 262.5753;
    fxc = 531.5340; fyc = 529.7583;
    
    LUT_x_steps = (x_fin-x_init)/x_inc +1;
    LUT_y_steps = (y_fin-y_init)/y_inc +1;
end
max_num_ipts = 100; %%%%% must be same for 'find_local_extrema', 'uc_to_xk' and 'ipts_to_3Dcolor'
num = max_num_ipts;

xk = zeros(1, num);
yk = zeros(1,num);
xn_c = zeros(4, num);

% convert ipts from (uc, vc) to (xk, yk)
for n = 1:num_pts

    xk(n) = (((2*double(ipts(2,n))) - uc0)/fxc); % image is 1/2 width
    yk(n) = ((2*double(ipts(1,n)+40)) - vc0)/fyc; % image is 1/2 height and cropped at row 40

% use LUT to convert (xk, yk) to (xn, yn)
    metricx = abs(xk_LUT(1,1,1)-xk(n));
    metricy = abs(xk_LUT(1,1,2)-yk(n));
    inx=1; jny=1;
    for i = 1:LUT_x_steps
        for j = 1:LUT_y_steps
            if abs(xk_LUT(j,i,1)-xk(n)) < metricx
                metricx = abs(xk_LUT(j,i,1)-xk(n));
                inx = i; % (xn, yn) indices from xk_LUT
            end
            if abs(xk_LUT(j,i,2)-yk(n)) < metricy
                metricy = abs(xk_LUT(j,i,2)-yk(n));
                jny = j; % (xn, yn) indicies from yk_LUT
            end
        end
    end
    % convert indices to metric
    xnx = x_init + (inx-1)*x_inc;
    yny = y_init + (jny-1)*y_inc;  
    % average values from xk_LUT and yk_LUT
    xn_c(:,n) = [(xnx); (yny); double(ipts(1,n)); double(ipts(2,n))];
      
end

== matlab function Find Interest Points in RGB/(ud,vd) to (xn,yn) ==
  data: d_cm input double; ipts_rpix input double; xn_d output double; xd_3D output double; max_depth input double; count output double
function [xn_d, xd_3D, count]  = d_to_xn(d_cm, ipts_rpix, max_depth)
% function converts all points in depth image into normalized color space (xn,yn)

% define persistent variables
persistent r11 r12 r13 r21 r22 r23 r33 t1 t2 ud0 vd0 fxd fyd
if isempty(r11)
    
    % Rrel from fabian_test_results_good.mat
    r11=0.9999; r12=-0.0071; r13=-0.0078;
    r21=0.0069; r22=0.9997; r23=-0.0240;
    r33= 0.9997; %%r31=0.0080; r32=0.0239;

    % Trel from fabian_test_results_good.mat
    t1=-2.08; t2=0.04; %%t3=0.06;

    % Depth camera intrinsics
    ud0 = 324.1963; vd0 = 232.6185;
    fxd = 590.4609; fyd = 582.7801;
end
%%%%%%%%%%%%%%%%%%%%%%%
max_num_ipts = 100;

% define ROI to search around each ipts
ROI = 10; % will create search area of (ROI+ROI+1)^2
%%%%%%%%%%%%%%%%%%%%%%%

array_size = (ROI+ROI+1)*(ROI+ROI+1);
xd_3D = zeros(array_size,max_num_ipts,3); % depth signal converted to 3D DEPTH coordinates
xn_d = zeros(array_size,max_num_ipts,2); % depth signal converted to NORMALIZED 3D COLOR coordinates

num_ipts = size(ipts_rpix,2);


count = zeros(1,max_num_ipts);
for n = 1:num_ipts
    % shorten variable names for convenience
    i_j = double(ipts_rpix(1,n));
    i_i = double(ipts_rpix(2,n));
    x=0; y=0; z=0;
    
    if i_i~=0 && i_j~=0
    for i = i_i-ROI:i_i+ROI
        for j = i_j-ROI:i_j+ROI
            count(n) = count(n) +1;
            if d_cm(j,i) <= max_depth && d_cm(j,i) ~=2848 % skip points further than 8m away
                
                z = double(d_cm(j,i));
                x = double((z/fxd)*(i*2 - ud0));
                y = double((z/fyd)*((j+40)*2 - vd0));
                xd_3D(count(n),n,1) = x; 
                xd_3D(count(n),n,2) = y; 
                xd_3D(count(n),n,3) = z;

                D = r33*z; % approximation based on relative size of terms in D
                xn_d(count(n),n,1) = (r11*x+r12*y+r13*z+t1)/D;
                xn_d(count(n),n,2) = (r21*x+r22*y+r23*z+t2)/D;

            end
        end
    end
    end
end

== matlab function Find Interest Points in RGB/3D Color Coord of ipts ==
  data: d_cm input double; xn_d input double; xd_3D input double; max_depth input double; num_pts input double; ipts_3D output double; ipts_dpix output double size=[2 100]; l1norm output double; xn_c input double; ipts_rpix output double size=[2 100]; x_offset input double; z_offset input double
function [ipts_3D, ipts_dpix, l1norm,ipts_rpix]  = ipts_to_3Ddepth(d_cm, xn_d,xd_3D, max_depth, num_pts, xn_c, x_offset, z_offset)
% function finds best match between ipts/xn from rgb and xn_d
% and generates 3D_DEPTH coordinates for each ipts


persistent ud0 vd0 fxd fyd
if isempty(ud0)
    % Depth camera intrinsics ('fabian_test_results_good.mat')
    ud0 = 324.1963; vd0 = 232.6185;
    fxd = 590.4609; fyd = 582.7801;
end

max_num_ipts = 100; %%%%% must be same for 'find_local_extrema', 'uc_to_xk' and 'ipts_to_3Dcolor'
dist_thres = 20; % threshold in pixels for match between ipts_rpix and ipts_dix
ROI = 10;
  
array_size = (ROI+ROI+1)*(ROI+ROI+1);

ipts_3D = zeros(3,max_num_ipts);
ipts_rpix=uint16(zeros(2,max_num_ipts));
ipts_rpix = uint16(xn_c(3:4,:));
ipts_dpix = uint16(zeros(2, max_num_ipts));
l1norm = 1;

% calculate L1norm between each pair of points in xn_d and xn_c
for i = 1:num_pts % loop over all ipts
    % get pix coord of current ipts
    xnx = xn_c(1,i);
    yny = xn_c(2,i);
    i_j = xn_c(3,i);
    i_i = xn_c(4,i);
    
    l1norm = (abs(xn_d(1,i,1)-xnx) + abs(xn_d(1,i,2)-yny));

    for c = 2:array_size
            if (abs(xn_d(c,i,1)-xnx) + abs(xn_d(c,i,2)-yny)) < l1norm 
                l1norm = (abs(xn_d(c,i,1)-xnx) + abs(xn_d(c,i,2)-yny)); 
                ipts_3D(:,i) = [xd_3D(c,i,1)+x_offset; xd_3D(c,i,2); xd_3D(c,i,3)+z_offset]; % adjust for offset of camera
                ipts_dpix(1,i) = uint16((((fyd*ipts_3D(2,i)/ipts_3D(3,i)) + vd0)/2)-40);
                ipts_dpix(2,i) = uint16((fxd*(ipts_3D(1,i)/ipts_3D(3,i)) + ud0)/2);
            end
    end
        
    % zero out bad matches
% %     if (abs(ipts_dpix(1,i)-i_j) + abs(ipts_dpix(2,i)-i_i)) > (dist_thres) ...
% %        || d_cm(ipts_dpix(1,i),ipts_dpix(2,i))>=max_depth
% %         ipts_dpix(:,i) = [0;0];
% %         ipts_rpix(:,i) = [0;0];
% %         ipts_3D(:,i) = [0;0;0];
% %     end
end

== matlab function Matching & Visodo/Feature Matching ==
  data: ipts_rpix input double; est_ipts input double; box input double; ipts input double; ipts_prev input double; M output double; num_cur input double; num_prev input double; num_match output double; miss_count output double; test output double; test2 output double; k input double; M_rpix output double
function [M, num_match, miss_count, test,test2, M_rpix] = feat_match(ipts_rpix,est_ipts, box, ipts, ipts_prev, num_cur, num_prev,k)


persistent miss 
if isempty(miss)
    miss=0; % 
end

max_num_ipts = 100; %%%%% must be same for 'find_local_extrema', 'uc_to_xk' and 'ipts_to_3Dcolor'

M = zeros(6,max_num_ipts);
M_rpix=uint16(zeros(2,max_num_ipts));
i = 0;
n=0;
same = 0;

% test = uint16(zeros(2,100));
test=zeros(4,100);
for c = 1:num_cur
    i=i+1;
    index = 0;
    metric = 1000;
    l1=zeros(1,100);
    y=ipts(2,c);
    x=ipts(1,c);
    z=ipts(3,c);
% %     test2=zeros(4,100);
    for p = 1:num_prev % loop through all est_ipts
        n=n+1;
        l1(1,p) = sum(abs(ipts(:,c)-est_ipts(:,p)));
        same = sum(ipts(:,c)-ipts_prev(:,p)); % =0 if they're the same
        
        xh=est_ipts(1,p);
        left=box(1,p);
        right=box(2,p);
        m=box(3,p);
        z2=box(4,p);
        z4=box(5,p);
        top_y=box(6,p);
        bot_y=box(7,p);
        
        back_z=m*(xh-right)+z2;
        front_z=m*(xh-right)+z4;
% %         test(1,p)=[l1(1,p)];
        if x>=left && x<=right && z<=back_z && z>=front_z && y<=top_y && y>=bot_y ...
                 && l1(1,p)<metric %&& same~=0
            index = index+1;
            metric = l1(1,p);
            M(1:3,i) = ipts_prev(:,p);
            M(4:6,i) = ipts(:,c); 
            M_rpix(:,i)=ipts_rpix(:,c);
            
        end
    end  % end prev
    [val,ind]=min(l1(1,1:num_prev));
    test(1:2,c)=[val;ind];
    if index ==0 % no matches found
        i=i-1; 
    end 
end  % end curr

num_match = i;
if num_match==0 % ie, no matches, use est_ipts
    miss=miss+1;
    M(1:3,1) = ipts_prev(:,1);
    M(4:6,1) = est_ipts(:,1);
end

miss_count = miss;
% outputs for testing
test2=zeros(6,100);
for p=1:num_prev
    xh=est_ipts(1,p);
    left=box(1,p);
    right=box(2,p);
    m=box(3,p);
    z2=box(4,p);
    z4=box(5,p);
    top_y=box(6,p);
    bot_y=box(7,p);

    back_z=m*(xh-right)+z2;
    front_z=m*(xh-right)+z4;
    test2(:,p)=[left;right;top_y;bot_y;back_z;front_z]
end

== matlab function Estimate Motion/ipts spacing ==
  data: ipts_3D input double; sigma output double; num_cur input double
function sigma  = spacing(ipts_3D, num_cur)
% function calculates distance to nearest ipts for each ipts in a single frame

persistent min_spacing_pers
if isempty(min_spacing_pers)
    min_spacing_pers=[0;0];
end

ipts = ipts_3D;
dist = zeros(1,99)+1000;
min_dist = zeros(1,100)+1000;
sigma=0;

for i=1:num_cur
    index = 0;
    if ipts(1,i)~=0
        for j=1:num_cur
            if j~=i && ipts(1,j)~=0
                index=index+1;
                dist(index) = sqrt((ipts(1,i)-ipts(1,j))^2 + (ipts(2,i)-ipts(2,j))^2 + (ipts(3,i)-ipts(3,j))^2);
            end
        end % j
    end
    min_dist(i) = min(dist); % closest neighbor for each ipts  

    if num_cur < 2
        min_dist(i)=min_spacing_pers(1,1);
    end
end % i

% % space = min(min_dist);
% % if space<min_spacing
% %     min_spacing=space
% % end
% % space=min_spacing;

% compute median of nearest neighbors
sigma = median(min_dist(1:num_cur));%std(min_dist(1:num_cur))];
min_spacing_pers(:,1) = sigma(:,1);

== matlab function Estimate Motion/Store ipts_prev ==
  data: ipts_prev output double; ipts_3D input double; ipts output double; num_cur output double; num_prev output double
function [ipts_prev, ipts, num_cur, num_prev] = store_ipts_prev(ipts_3D)
% function takes ipts_3D and stores ipts_prev, also returns num_cur and num_prev


max_num_ipts = 100; %%%%% must be same for 'find_local_extrema', 'uc_to_xk' and 'ipts_to_3Dcolor'

persistent ipts_prev_pers num_prev_pers

if isempty(ipts_prev_pers)
    ipts_prev_pers = ipts_3D;
    num_prev_pers = 0;
end

num_cur = 0;
num_prev = num_prev_pers;
ipts = zeros(3,max_num_ipts);
ipts_prev = ipts_prev_pers;

for i=1:size(ipts_3D,2)
    if ipts_3D(3,i) ~= 0
        num_cur = num_cur+1;
        ipts(:,num_cur) = ipts_3D(:,i);
    end
end

ipts_prev_pers = ipts;
num_prev_pers = num_cur;
